simulink library "Limiter"  (R2022b)
settings: Solver=VariableStepAuto  StartTime=0.0  StopTime=10.0  RelTol=1e-3
libraries: LimiterBtc x1
settings Model: Creator=jb10849  LastModifiedBy=kl13806
settings SolverCC: AlgebraicLoopSolver=TrustRegion
settings DebuggingCC: UnconnectedInputMsg=warning  UnconnectedOutputMsg=warning  UnconnectedLineMsg=warning  SFMachineParentedDataDiag=warning  ArithmeticOperatorsInVariantConditions=warning
settings ModelReferenceCC: EnableRefExpFcnMdlSchedulingChecks=on
settings SFSimCC: SimUseLocalCustomCode=off  CustomCodeUndefinedFunction=UseInterfaceOnly
settings RTWCC: RTWUseLocalCustomCode=off  DLArmComputeVersion=19.05

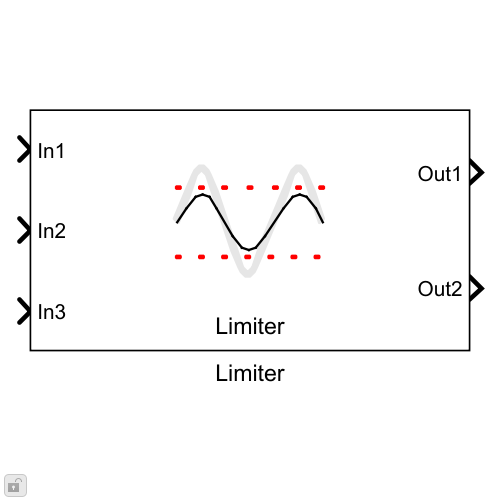
[thumbnail: Simulink's stored preview of the top-level diagram]
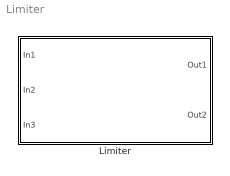
== system Limiter ==
  Limiter : Subsystem  mask{attackDB=[], decayDB=[], maxAttackTuningValue=[], threshold=[], attackDB_low=[], decayDB_low=[], maxAttack_low=[], threshold_low=[]}
      mask prompts: attackDB "Attack in dB"; decayDB "Decay in dB"; maxAttackTuningValue "MaxAttack"; attackDB_low "Attack (low) in dB"; decayDB_low "Decay (low) in dB"; maxAttack_low "Max Attack (low)"; threshold_low "Threshold (low)"
      mask init:
      | blkh = gcbh;
      | % Copy discrete mask parameters into a classdef object
      | InnerLinkConfig = LimiterConfig;
      | InnerLinkConfig.DefaultAttackDb = attackDB;
      | InnerLinkConfig.DefaultDecayDB = decayDB;
      | InnerLinkConfig.DefaultMaxAttackDb = maxAttackTuningValue;
      | InnerLinkConfig.DefaultThreshold = threshold;
      | InnerLinkConfig.DefaultAttackLowDb = attackDB_low;
      | InnerLinkConfig.DefaultDecayLowDb = decayDB_low;
      | InnerLinkConfig.DefaultMaxAttackLowDb = maxAttack_low;
      | InnerLinkConfig.DefaultThresholdLow = threshold_low;
      mask DialogControl Container3 Prompt: Parameter Set 1
      mask DialogControl Container4 Prompt: Parameter Set 2 (for start-stop situation)
      mask Display:
      | [path,w,h] = IconLimiterMask();
      | 
      | % work in pixels since the icon does not scale
      | pos = get(gcbh,'position');
      | bw = pos(3) - pos(1);
      | bh = pos(4) - pos(2);
      | 
      | % Draw centered icon
      | xAdj = bw/2 - w/2;
      | yAdj = bh/2 - h/2 + 4;
      | for i=1:length(path)
      |     if (path(i).rgb(1) >= 0)
      |         patch(path(i).x+xAdj, path(i).y+yAdj, path(i).rgb);
      |     end
      |     if (path(i).stroke(1) >= 0)
      |         plot(path(i).x+xAdj, path(i).y+yAdj);
      |     end
      | end
      | 
      | % Anchor the corners of the coordinate system
      | patch(0,0,[1 1 1]);
      | patch(bw,bh,[1 1 1]);
      | 
      | % Display some text
      | text(bw/2, 4,'Limiter', ...
      |     'horizontalAlignment','center', ...
      |     'VerticalAlignment','bottom');

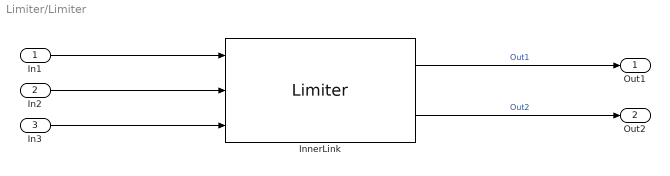
== system Limiter/Limiter ==
  In1 : Inport
  In2 : Inport  Port=2
  In3 : Inport  Port=3
  InnerLink : LimiterBtc/Limiter  Config=InnerLinkConfig  FeatureName=Limiter
      settings: SourceProductName=Bose Blocklib
  Out1 : Outport
  Out2 : Outport  Port=2
  wires:
  InnerLink/1 -> Out1/1  "Out1"
  InnerLink/2 -> Out2/1  "Out2"
  In1/1 -> InnerLink/1
  In2/1 -> InnerLink/2
  In3/1 -> InnerLink/3
